simulink model "ex_inverter_single_full_bridge_unipoPWM_vs_bipoPWM"  (R2022b)
settings: Solver=VariableStepAuto  StartTime=0.0  StopTime=0.1  RelTol=1e-3
libraries: spsMosfetLib x8, spsDCVoltageSourceLib x4, spsFourierLib x4, spsVoltageMeasurementLib x2, spsGroundLib x2, spsMultimeterLib x2, spsRMSLib x2, simulink x2, spsSeriesRLCBranchLib x2, spsTHDLib x2, sps_lib x1
settings Model: Creator=realj  LastModifiedBy=realj

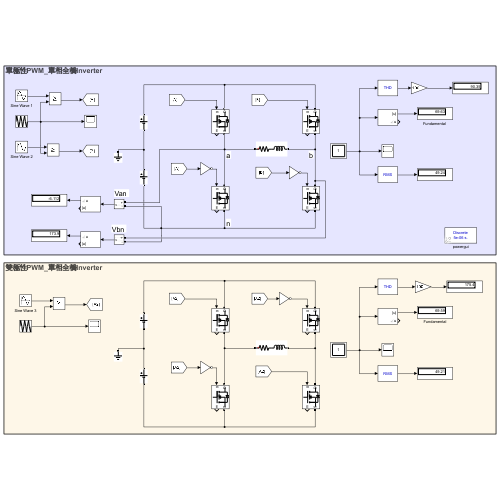
[thumbnail: Simulink's stored preview of the top-level diagram]
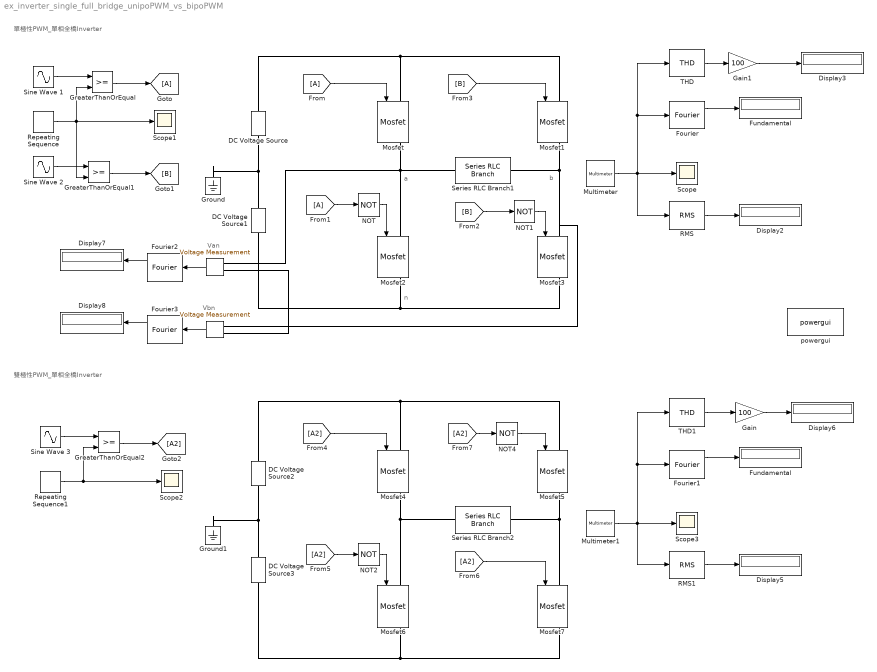
== system ex_inverter_single_full_bridge_unipoPWM_vs_bipoPWM ==
  note: a
  note: 雙極性PWM_單相全橋Inverter
  note: 單極性PWM_單相全橋Inverter
  note: b
  note: n
  note: Van
  note: Vbn
  " " : spsVoltageMeasurementLib/Voltage Measurement  PhasorSimulation=off  OutputType=Complex  PSBequivalent=0
  "  " : spsVoltageMeasurementLib/Voltage Measurement  PhasorSimulation=off  OutputType=Complex  PSBequivalent=0
  DC Voltage Source{,1..3} (4 alike) : spsDCVoltageSourceLib/DC Voltage Source  Amplitude=50  Measurements=None
  Display{2..3,5..8} (6 alike) : Display
  Fourier : spsFourierLib/Fourier  Freq=50  n=1  InInit=[0, 0]  Ts=0
  Fourier1 : spsFourierLib/Fourier  Freq=50  n=1  InInit=[0, 0]  Ts=0
  Fourier2 : spsFourierLib/Fourier  Freq=50  n=49  InInit=[0, 0]  Ts=0
  Fourier3 : spsFourierLib/Fourier  Freq=50  n=49  InInit=[0, 0]  Ts=0
  From : From
  From1 : From
  Fundamental : Display
  "Fundamental " : Display
  Gain : Gain  Gain=100
  Gain1 : Gain  Gain=100
  Goto : Goto
  GreaterThanOrEqual : RelationalOperator  OutDataTypeStr=boolean  RndMeth=Simplest  InputSameDT=off
  GreaterThanOrEqual1 : RelationalOperator  OutDataTypeStr=boolean  RndMeth=Simplest  InputSameDT=off
  GreaterThanOrEqual2 : RelationalOperator  OutDataTypeStr=boolean  RndMeth=Simplest  InputSameDT=off
  Ground : spsGroundLib/Ground  LConnTagsString=a
  Ground1 : spsGroundLib/Ground  LConnTagsString=a
  Mosfet{,1..7} (8 alike) : spsMosfetLib/Mosfet  Ron=0.1  Lon=0  Rd=0.01  Vfd=0  IC=0  Rs=1e5  Cs=inf  Measurements=on
  Multimeter : spsMultimeterLib/Multimeter  L=2  sel=1  yselected={}  Gain=1  OutputType=Complex  PlotAtSimulationStop=off  PhasorSimulation=off
  Multimeter1 : spsMultimeterLib/Multimeter  L=2  sel=2  yselected={}  Gain=1  OutputType=Complex  PlotAtSimulationStop=off  PhasorSimulation=off
  NOT{,1..2,4} (4 alike) : Logic  Operator=NOT  IconShape=distinctive  AllPortsSameDT=off  OutDataTypeStr=boolean
  RMS : spsRMSLib/RMS  TrueRMS=off  Freq=50  RMSInit=0  Ts=0
  RMS1 : spsRMSLib/RMS  TrueRMS=off  Freq=50  RMSInit=0  Ts=0
  Repeating Sequence : simulink/Sources/Repeating Sequence  rep_seq_t=[0 1 2 3 4]*1/(24*50*4)  rep_seq_y=[0 1 0 -1 0]
  Repeating Sequence1 : simulink/Sources/Repeating Sequence  rep_seq_t=[0 1 2 3 4]*1/(24*50*4)  rep_seq_y=[0 1 0 -1 0]
  Scope{,1..3} (4 alike) : Scope
  Series RLC Branch1 : spsSeriesRLCBranchLib/Series RLC Branch  LConnTagsString=__new0  RConnTagsString=__new0  BranchType=RL  Resistance=25  Inductance=1e-3  SetiL0=off  InitialCurrent=0  Capacitance=1e-6  Setx0=off  InitialVoltage=0  Measurements=Branch voltage
  Series RLC Branch2 : spsSeriesRLCBranchLib/Series RLC Branch  LConnTagsString=__new0  RConnTagsString=__new0  BranchType=RL  Resistance=25  Inductance=1e-3  SetiL0=off  InitialCurrent=0  Capacitance=1e-6  Setx0=off  InitialVoltage=0  Measurements=Branch voltage
  Sine Wave 1 : Sin  Amplitude=.7  Frequency=2*pi*50  SampleTime=0
  Sine Wave 2 : Sin  Amplitude=.7  Frequency=2*pi*50  Phase=pi  SampleTime=0
  Sine Wave 3 : Sin  Amplitude=.7  Frequency=2*pi*50  SampleTime=0
  THD : spsTHDLib/THD  Freq=50  Ts=0
  THD1 : spsTHDLib/THD  Freq=50  Ts=0
  powergui : sps_lib/powergui  Priority=1  SimulationMode=Discrete  SampleTime=5e-6  frequency=60  Iterations=50  frequencyindice=0  Pbase=100e6  ErrMax=1e-4  UnitsV=kV  UnitsW=MW  buscounter=0  FunctionMessages=off  echomessages=off  EnableUseOfTLC=off  CurrentSourceSwitches=off  DisableSnubberDevices=off  DisableRonSwitches=off  DisableVfSwitches=off  DisplayEquations=off  AutomaticDiscreteSolvers=off  SolverType=Tustin/Backward Euler (TBE)  Interpol=off  ExternalGateDelay=off  methode=off  Ts=100  x0status=blocks  SPID=on  SwTol=0  HookPort=off  NonlinearTolerance=1e-4  nMaxIteration=100  ContinueOnMaxIteration=off  RestoreLinks=warning  ResistiveCurrentMeasurement=off  Frange=[0:2:500]  Ylog=off  Xlog=on  ShowGrid=off  save=off  variable=ZData  structure=0  ZoomFFT=off  StartTime=0.0  cycles=1  DisplayStyle=1  fundamental=60  FreqAxis=off  MaxFrequency=1000  frequencyindicesteady=1  RmsSteady=1  display=off
  wires:
  Sine Wave 1/1 -> GreaterThanOrEqual/1
  Repeating Sequence/1 -> GreaterThanOrEqual1/2, Scope1/1, GreaterThanOrEqual/2
  Sine Wave 2/1 -> GreaterThanOrEqual1/1
  GreaterThanOrEqual/1 -> Goto/1
  GreaterThanOrEqual1/1 -> [B]
  From/1 -> Mosfet/1
  From1/1 -> NOT/1
  NOT/1 -> Mosfet2/1
  NOT1/1 -> Mosfet3/1
  [B] -> NOT1/1
  [B] -> Mosfet1/1
  RMS/1 -> Display2/1
  Fourier/1 -> "Fundamental "/1
  THD/1 -> Gain1/1
  Multimeter/1 -> RMS/1, Fourier/1, THD/1, Scope/1
  GreaterThanOrEqual2/1 -> [A2]
  Repeating Sequence1/1 -> GreaterThanOrEqual2/2, Scope2/1
  Sine Wave 3/1 -> GreaterThanOrEqual2/1
  Multimeter1/1 -> Scope3/1, THD1/1, Fourier1/1, RMS1/1
  Fourier1/1 -> Fundamental/1
  RMS1/1 -> Display5/1
  [A2] -> NOT4/1
  [A2] -> Mosfet7/1
  NOT2/1 -> Mosfet6/1
  [A2] -> NOT2/1
  [A2] -> Mosfet4/1
  NOT4/1 -> Mosfet5/1
  THD1/1 -> Gain/1
  " "/1 -> Fourier2/1
  "  "/1 -> Fourier3/1
  Fourier2/2 -> Display7/1
  Fourier3/2 -> Display8/1
  Gain/1 -> Display6/1
  Gain1/1 -> Display3/1
  connections:
  Series RLC Branch1/RConn1 -- "  "/LConn1 -- Mosfet3/LConn1 -- Mosfet1/RConn1
  Series RLC Branch1/LConn1 -- Mosfet/RConn1 -- " "/LConn1 -- Mosfet2/LConn1
  DC Voltage Source/RConn1 -- Mosfet1/LConn1 -- Mosfet/LConn1
  Mosfet2/RConn1 -- "  "/LConn2 -- " "/LConn2 -- DC Voltage Source1/LConn1 -- Mosfet3/RConn1
  DC Voltage Source1/RConn1 -- Ground/LConn1 -- DC Voltage Source/LConn1
  Series RLC Branch2/RConn1 -- Mosfet5/RConn1 -- Mosfet7/LConn1
  Series RLC Branch2/LConn1 -- Mosfet4/RConn1 -- Mosfet6/LConn1
  DC Voltage Source2/RConn1 -- Mosfet5/LConn1 -- Mosfet4/LConn1
  Mosfet6/RConn1 -- DC Voltage Source3/LConn1 -- Mosfet7/RConn1
  DC Voltage Source3/RConn1 -- DC Voltage Source2/LConn1 -- Ground1/LConn1
